simulink model "TFlex_I_FITC"  (R2018a)
settings: Solver=VariableStepAuto  StartTime=0.0  StopTime=10.0  RelTol=1e-3
undefined symbols (not defined in the file): a0, a1, a2, Avout, b, D, DiscIntNeverNeededParam, FB1_offset, h, hyp, I_limit_max, I_limit_min, Kd, Ki, Kp, kp, KTY_p0, KTY_p1, Kuu, LPden, LPnum, Lu, mu_u, Nkeep, R, r, seed, sf, SIGMA, sn, sp_ts, tau_i, tau_p, tau_z, tm, ts, var_u, w
libraries: xpcethercatlib x17, simulink x10, dspindex x6, slrtlib x5, dspfactors x2, dspmtrx3 x2
(part 2 of 2)

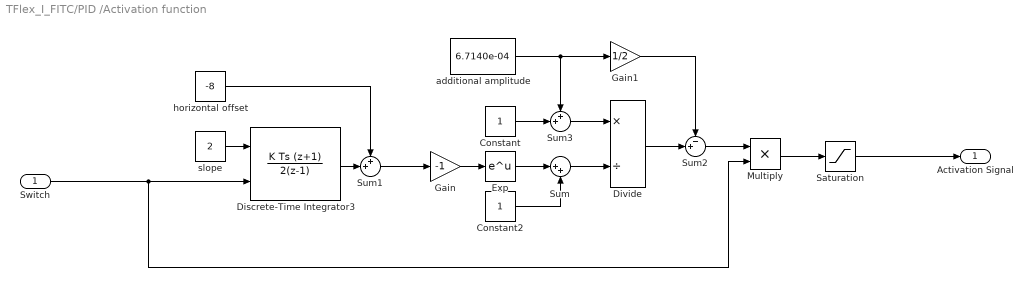
== system TFlex_I_FITC/PID /Activation function ==
  Switch : Inport
  Constant : Constant
  Constant2 : Constant
  Discrete-Time Integrator3 : DiscreteIntegrator  IntegratorMethod=Integration: Trapezoidal  ExternalReset=rising  SampleTime=-1  UpperSaturationLimit=1  LowerSaturationLimit=0  ICPrevOutput=DiscIntNeverNeededParam  ICPrevScaledInput=DiscIntNeverNeededParam
  Divide : Product  Inputs=*/
  Exp : Math  SaturateOnIntegerOverflow=on
  Gain : Gain  Gain=-1
  Gain1 : Gain  Gain=1/2
  Multiply : Product
  Saturation : Saturate  UpperLimit=1  LowerLimit=0
  Sum : Sum  Inputs=|++
  Sum1 : Sum  Inputs=++|
  Sum2 : Sum  Inputs=-+|
  Sum3 : Sum  Inputs=++|
  additional amplitude : Constant  Value=6.7140e-04
  horizontal offset : Constant  Value=-8
  slope : Constant  Value=2
  Activation Signal : Outport
  wires:
  Constant/1 -> Sum3/2
  Exp/1 -> Sum/1
  additional amplitude/1 -> Sum3/1, Gain1/1
  Sum1/1 -> Gain/1
  Gain1/1 -> Sum2/1
  Divide/1 -> Sum2/2
  Sum/1 -> Divide/2
  Gain/1 -> Exp/1
  slope/1 -> Discrete-Time Integrator3/1
  Discrete-Time Integrator3/1 -> Sum1/2
  Constant2/1 -> Sum/2
  Sum2/1 -> Multiply/1
  Sum3/1 -> Divide/1
  horizontal offset/1 -> Sum1/1
  Saturation/1 -> Activation Signal/1
  Multiply/1 -> Saturation/1
  Switch/1 -> Multiply/2, Discrete-Time Integrator3/2

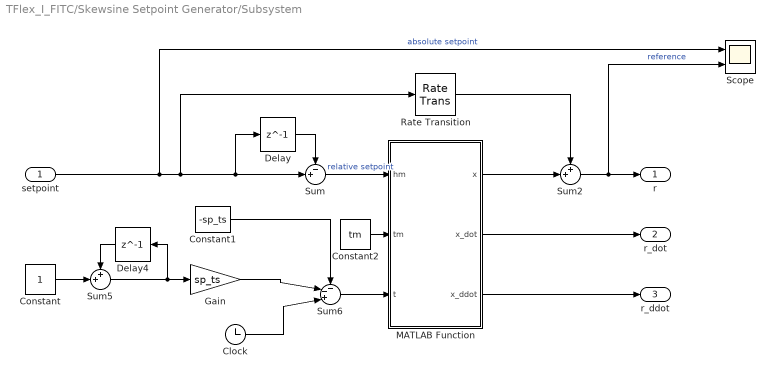
== system TFlex_I_FITC/Skewsine Setpoint Generator/Subsystem ==
  setpoint : Inport
  Clock : Clock
      settings: Decimation=100
  Constant : Constant  SampleTime=sp_ts
  Constant1 : Constant  Value=-sp_ts  SampleTime=sp_ts
  Constant2 : Constant  Value=tm  SampleTime=sp_ts
  Delay : Delay  DelayLength=1  InitialCondition=0  SampleTime=sp_ts
  Delay4 : Delay  DelayLength=1  InitialCondition=0  SampleTime=sp_ts
  Gain : Gain  Gain=sp_ts
  MATLAB Function : MATLAB Function  TreatAsAtomicUnit=on
  Rate Transition : RateTransition  OutPortSampleTime=ts
  Scope : Scope  NumInputPorts=2
  Sum : Sum  Inputs=-+|
  Sum2 : Sum  Inputs=++|
  Sum5 : Sum  Inputs=++|
  Sum6 : Sum  Inputs=--+|
  r : Outport
  r_dot : Outport  Port=2
  r_ddot : Outport  Port=3
  wires:
  Delay4/1 -> Sum5/1
  Sum2/1 -> r/1, Scope/2  "reference"
  Sum5/1 -> Delay4/1, Gain/1
  Constant/1 -> Sum5/2
  MATLAB Function/3(x_ddot) -> r_ddot/1
  Clock/1 -> Sum6/3
  Delay/1 -> Sum/1
  Gain/1 -> Sum6/2
  Constant1/1 -> Sum6/1
  MATLAB Function/2(x_dot) -> r_dot/1
  Sum/1 -> MATLAB Function/1(hm)  "relative setpoint"
  Constant2/1 -> MATLAB Function/2(tm)
  Sum6/1 -> MATLAB Function/3(t)
  MATLAB Function/1(x) -> Sum2/2
  setpoint/1 -> Scope/1, Rate Transition/1, Delay/1, Sum/2  "absolute setpoint"
  Rate Transition/1 -> Sum2/1

== system TFlex_I_FITC/Update Posterior/Features ==
  x : Inport
  SIGMA : Inport  Port=2
  sf : Inport  Port=3
  D : Inport  Port=4
  Divide2 : Product  Inputs=*/
  Product : Product  Multiplication=Matrix(*)
  Product2 : Product
  Sqrt : Sqrt  SaturateOnIntegerOverflow=on
  Transpose2 : Math  Operator=transpose  SaturateOnIntegerOverflow=on
  Transpose3 : Math  Operator=transpose  SaturateOnIntegerOverflow=on
  Transpose4 : Math  Operator=transpose  SaturateOnIntegerOverflow=on
  Trigonometric Function : Trigonometry  Operator=cos
  Trigonometric Function1 : Trigonometry
  Vector Concatenate1 : Concatenate
  phi_out : Outport
  wires:
  SIGMA/1 -> Product/1
  Product2/1 -> phi_out/1
  D/1 -> Sqrt/1
  Trigonometric Function1/1 -> Transpose3/1
  Trigonometric Function/1 -> Transpose2/1
  sf/1 -> Divide2/1
  Vector Concatenate1/1 -> Transpose4/1
  Transpose3/1 -> Vector Concatenate1/2
  Product/1 -> Trigonometric Function1/1, Trigonometric Function/1
  Divide2/1 -> Product2/1
  Transpose4/1 -> Product2/2
  Sqrt/1 -> Divide2/2
  Transpose2/1 -> Vector Concatenate1/1
  x/1 -> Product/2

== stateflow chart TFlex_I_FITC/Chart2 ==
  state ON
    Y=0;
  state OFF
    Y=0;
  state OFF1
    Y=u;
  (default) -> ON
  ON -> OFF : [u<90]
  OFF -> OFF1 [order 2] : [t>10]
  OFF -> ON [order 1] : [u>90]
  OFF1 -> OFF : [u>90]
  data: u input; Y output; t input

== matlab function TFlex_I_FITC/Update Posterior/MATLAB Function ==
  settings: updateMethod=DISCRETE  sampleTime=ts
  data: R input; w_out output; b input; w_init input
function w_out = updateW(R,b,w_init)
persistent w
if(isempty(w))
    w = w_init;
end
%coder.extrinsic('solve_chol');
%w = solve_chol(R,b);
w = R\(R'\b);
w_out = w;

== matlab function TFlex_I_FITC/Skewsine Setpoint Generator/Subsystem/MATLAB Function ==
  settings: updateMethod=DISCRETE  sampleTime=ts
  data: hm input; x output; tm input; t input; x_dot output; x_ddot output
function [x,x_dot,x_ddot] = skewSine(hm,tm,t)

if (t>=0) && (t<=tm)
    x      = hm/tm*t - hm/(2*pi)*sin(2*pi/tm*t);
    x_dot  = hm/tm - hm/tm*cos(2*pi/tm*t);
    x_ddot = 2*pi*hm/(tm^2)*sin(2*pi/tm*t);
else
    x      = hm;
    x_dot  = 0;
    x_ddot = 0;
end

== stateflow chart TFlex_I_FITC/Chart1 ==
  state OFF2
    Y=0;
  state ON
    Y=u;
  (default) -> OFF2
  OFF2 -> ON : [t>10]
  ON -> OFF2 : [t<10]
  data: u input; Y output; t input

== matlab function TFlex_I_FITC/MATLAB Function1 ==
  data: hyp input; sn input; u input; u output; mu_u input; var_u input; Kuu input; uNew input size=[1,3]; Kuu output; Lu output; mu_u output; var_u output
function [u,Kuu,Lu,mu_u,var_u] = uUpdate(hyp,sn,u,mu_u,var_u,Kuu,uNew)%#codegen
coder.extrinsic('updateInducing');
Lu = double(zeros(size(Kuu)));
[u,Kuu,Lu,mu_u,var_u,Mu] = updateInducing(hyp,sn,u,mu_u,var_u,Kuu,uNew,0);

== matlab function TFlex_I_FITC/Update Posterior/MATLAB Function1 ==
  settings: updateMethod=DISCRETE  sampleTime=ts
  data: R_out output; phi input; R_init input
function R_out = cholupdate_fcn(phi,R_init)
persistent R; 
if(isempty(R))
    R = R_init;
end
R = cholupdate(R,phi);
R_out = R;

== matlab function TFlex_I_FITC/Transient Setpoint Generator2/MATLAB Function2 ==
  data: v1 input; output output; v2 input; r0 input; h0 input
function output = Fhan(v1,v2,r0, h0)
d = h0^2*r0;
a0 = h0*v2;
y = v1 + a0;
a1 = sqrt(d*(d+8*abs(y)));
a2 = a0 + sign(y)*(a1-d)/2;
sy = (sign(y+d)-sign(y-d))/2;
a = (a0+y-a2)*sy +a2;
sa = (sign(a+d)-sign(a-d))/2;
output = -r0 *(a/d -sign(a) )*sa - r0*sign(a);

== matlab function TFlex_I_FITC/Update Posterior/MATLAB Function4 ==
  settings: updateMethod=DISCRETE  sampleTime=ts
  data: update input; b_out output; b_init input
function b_out = updateB(update, b_init)
persistent b 
if(isempty(b))
    b = b_init;
end

b = b + update;
b_out = b;

== matlab function TFlex_I_FITC/Subsystem1/Kuup_n ==
  data: x1 input; K output size=[Nkeep+1,Nkeep+1]; x2 input; hyp input
function K = SquaredExpCov(x1,x2,hyp) %#codegen
coder.extrinsic('SEcov');
n = size(x1,1);
K = double(zeros(n));
K = SEcov(x1,x2,hyp);
end

== matlab function TFlex_I_FITC/Subsystem1/Kuup_n1 ==
  data: x1 input; K output size=[Nkeep,1]; x2 input; hyp input
function K = SquaredExpCov(x1,x2,hyp) %#codegen
coder.extrinsic('SEcov');
n = size(x1,1);
K = double(zeros(n,1));
K = SEcov(x1,x2,hyp);
end

== matlab function TFlex_I_FITC/Subsystem1/Kuup_n2 ==
  data: x1 input; K output size=[1,1]; x2 input; hyp input
function K = SquaredExpCov(x1,x2,hyp) %#codegen
coder.extrinsic('SEcov');
K = double(1);
K = SEcov(x1,x2,hyp);
end

== matlab function TFlex_I_FITC/MATLAB Function ==
  data: mu_u output; var_u output; hyp input size=[1,4]; sn input size=1; fp input size=[1,3]; yfp input size=[1]; mu_u input size=[Nkeep+1,1]; var_u input; u input; Lu input; Kuu input; mu output size=1; sNew input size=[1,3]
function [mu_u,var_u,mu] = I_FITC(hyp,sn,fp,yfp,mu_u,var_u,u,Lu,Kuu,sNew) %#codegen
coder.extrinsic('IncrementalFITC');
mu = double(1);
[mu, var ,mu_u,var_u] = IncrementalFITC(hyp,sn,u,sNew,fp,yfp,mu_u,var_u,Lu,Kuu);

== matlab function TFlex_I_FITC/Subsystem2/K_uu  ==
  data: x1 input size=[1,3]; K output size=[1,1]; x2 input size=[1,3]; hyp input
function K = SquaredExpCov(x1,x2,hyp) %#codegen
coder.extrinsic('SEcov');
n = size(x1,1);
K = double(zeros(n,1));
K = SEcov(x1,x2,hyp);
end

== matlab function TFlex_I_FITC/Subsystem2/K_uu 1 ==
  data: x1 input; K output size=[Nkeep+1,1]; x2 input; hyp input
function K = SquaredExpCov(x1,x2,hyp) %#codegen
coder.extrinsic('SEcov');
n = size(x1,1);
K = double(zeros(n,1));
K = SEcov(x1,x2,hyp);
end

== matlab function TFlex_I_FITC/Subsystem2/K_uu 2 ==
  data: x1 input; K output size=[1,1]; x2 input; hyp input
function K = SquaredExpCov(x1,x2,hyp) %#codegen
coder.extrinsic('SEcov');
n = size(x1,1);
K = double(zeros(n,1));
K = SEcov(x1,x2,hyp);
end

== matlab function TFlex_I_FITC/Subsystem2/K_uu 3 ==
  data: x1 input; K output size=[Nkeep+1,1]; x2 input; hyp input
function K = SquaredExpCov(x1,x2,hyp) %#codegen
coder.extrinsic('SEcov');
n = size(x1,1);
K = double(zeros(n,1));
K = SEcov(x1,x2,hyp);
end

== matlab function TFlex_I_FITC/Subsystem2/MATLAB Function ==
  data: Lu input; Lu_inv output
function Lu_inv = inverse(Lu)
Lu_inv = inv(Lu);

== matlab function TFlex_I_FITC/Subsystem2/MATLAB Function1 ==
  data: u input; y output
function y = Trace(u)
y = trace(u);

== matlab function TFlex_I_FITC/Subsystem2/MATLAB Function3 ==
  data: u input; y output
function y = Trace(u)
y = trace(u);
